simulink model "KalmanFIlter"  (R2022b)
settings: Solver=VariableStepAuto  StartTime=0.0  StopTime=timetorevolve  RelTol=1e-3
model workspace (MAT data in the model file):
  Ts_Camera = 0.1
values from neighbouring files (symbols this model uses):
  ConstantO = 2*pi/(timetorevolve)    (= 0.00118999721727)    [SystemVariables.m]
  Ts_System = 1/system_Frequency    (= 0.1)    [SystemVariables.m]
libraries: robotcorelib x3, simulink x1
settings Model: Creator=Xamza  LastModifiedBy=Xamza

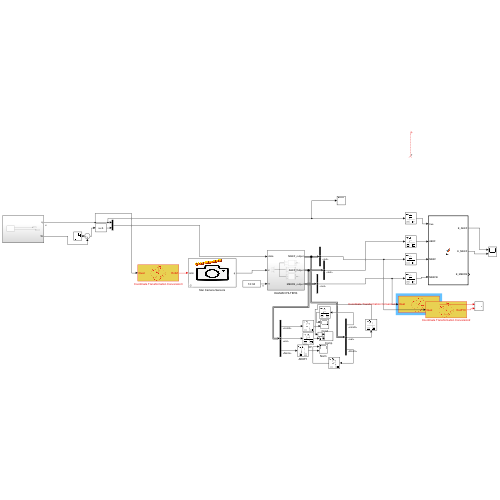
[thumbnail: Simulink's stored preview of the top-level diagram]
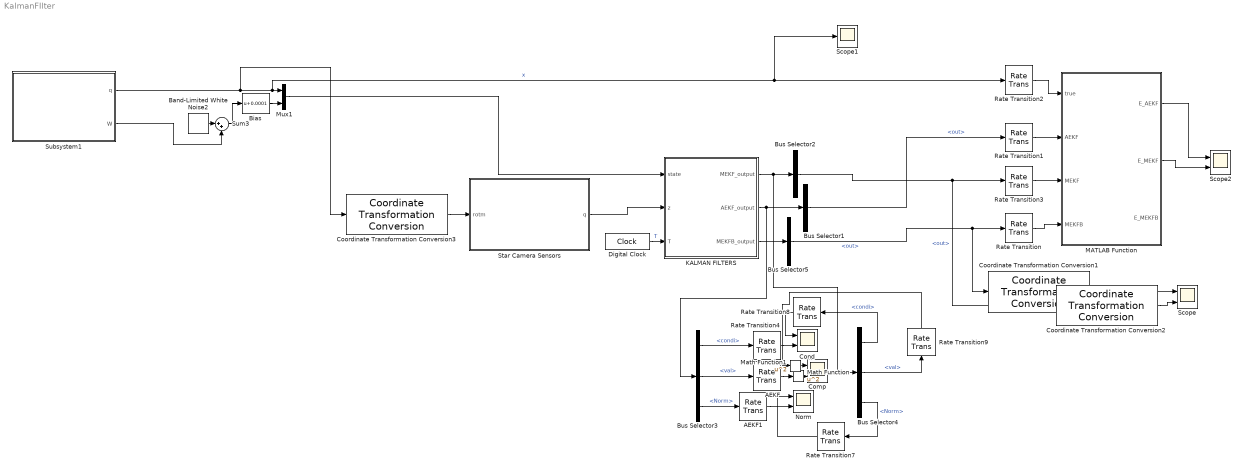
== system KalmanFIlter ==
  AEKF : RateTransition  Integrity=off  OutPortSampleTime=ComTs
  AEKF1 : RateTransition  Integrity=off  OutPortSampleTime=ComTs
  Band-Limited White Noise2 : simulink/Sources/Band-Limited White Noise  Cov=[0.00001]  Ts=Ts_System  seed=[23341]
  Bias : Bias  Bias=0.0001  SaturateOnIntegerOverflow=off
  Bus Selector1 : BusSelector  OutputSignals=out
  Bus Selector2 : BusSelector  OutputSignals=out
  Bus Selector3 : BusSelector  OutputSignals=condi,val,Norm
  Bus Selector4 : BusSelector  OutputSignals=condi,val,Norm
  Bus Selector5 : BusSelector  OutputSignals=out
  Comp : Scope  NumInputPorts=2
  Cond : Scope  NumInputPorts=2
  Coordinate Transformation Conversion1 : robotcorelib/Coordinate Transformation Conversion  InputRepresentation=Quaternion  InputEulerSequence=ZYX  ShowTrVecInputPort=on  OutputRepresentation=Euler Angles  OutputEulerSequence=ZYX  ShowTrVecOutputPort=on  SimulateUsing=Interpreted execution
  Coordinate Transformation Conversion2 : robotcorelib/Coordinate Transformation Conversion  InputRepresentation=Quaternion  InputEulerSequence=ZYX  ShowTrVecInputPort=on  OutputRepresentation=Euler Angles  OutputEulerSequence=ZYX  ShowTrVecOutputPort=on  SimulateUsing=Interpreted execution
  Coordinate Transformation Conversion3 : robotcorelib/Coordinate Transformation Conversion  InputRepresentation=Quaternion  InputEulerSequence=ZYX  ShowTrVecInputPort=on  OutputRepresentation=Rotation Matrix  OutputEulerSequence=ZYX  ShowTrVecOutputPort=on  SimulateUsing=Interpreted execution
  Digital Clock : DigitalClock  SampleTime=Ts_System
  KALMAN FILTERS : Subsystem
  MATLAB Function : MATLAB Function  TreatAsAtomicUnit=on
  Math Function : Math  Operator=square
  Math Function1 : Math  Operator=square
  Mux1 : Mux  Inputs=2
  Norm : Scope  NumInputPorts=2
  Rate Transition{,1..4,7..9} (8 alike) : RateTransition  Integrity=off  OutPortSampleTime=ComTs
  Scope : Scope  NumInputPorts=2
  Scope1 : Scope
  Scope2 : Scope  NumInputPorts=2
  Star Camera Sensors : Subsystem  mask{StarOne=on, StarTwo=on, StarThree=on, StarFour=on, StarFive=on, StarSix=on}
      mask prompts: StarOne "Star Camera One"; StarTwo "Star Camera Two"; StarThree "Star Camera Three"; StarFour "Star Camera Four"; StarFive "Star Camera Five"; StarSix "Star Camera Six"
      mask DialogControl DescGroupVar Prompt: Star Camera Settings
      mask DialogControl ParameterGroupVar Prompt: Available Star Cameras
      mask Display: image('$imagefile'); % Use "Edit Image" on toolstrip to change.
  Subsystem1 : Subsystem
  Sum3 : Sum  Inputs=|++
  wires:
  Coordinate Transformation Conversion3/1 -> Star Camera Sensors/1(rotm)
  Star Camera Sensors/1(q) -> KALMAN FILTERS/2(z)
  ? -> ?  "T"
  Sum3/1 -> Bias/1
  Subsystem1/1(q) -> Scope1/1, Rate Transition2/1, Mux1/1, Coordinate Transformation Conversion3/1  "x"
  Subsystem1/2(W) -> Sum3/2
  Band-Limited White Noise2/1 -> Sum3/1
  MATLAB Function/1(E_AEKF) -> Scope2/1
  MATLAB Function/2(E_MEKF) -> Scope2/2
  Rate Transition/1 -> MATLAB Function/4(MEKFB)
  Rate Transition1/1 -> MATLAB Function/2(AEKF)
  Rate Transition2/1 -> MATLAB Function/1(true)
  Mux1/1 -> KALMAN FILTERS/1(state)
  Digital Clock/1 -> KALMAN FILTERS/3(T)  "T"
  KALMAN FILTERS/2(AEKF_output) -> Bus Selector3/1, Bus Selector1/1
  KALMAN FILTERS/3(MEKFB_output) -> Bus Selector5/1
  Bus Selector3/1 -> Rate Transition4/1  "<condi>"
  Bus Selector3/3 -> AEKF1/1  "<Norm>"
  Bus Selector3/2 -> AEKF/1  "<val>"
  KALMAN FILTERS/1(MEKF_output) -> Bus Selector2/1, Bus Selector4/1
  Bus Selector4/1 -> Rate Transition8/1  "<condi>"
  Bus Selector4/2 -> Rate Transition9/1  "<val>"
  Bus Selector4/3 -> Rate Transition7/1  "<Norm>"
  Bias/1 -> Mux1/2
  Bus Selector5/1 -> Rate Transition/1, Coordinate Transformation Conversion1/1  "<out>"
  Rate Transition3/1 -> MATLAB Function/3(MEKF)
  Bus Selector1/1 -> Rate Transition1/1  "<out>"
  Bus Selector2/1 -> Rate Transition3/1, Coordinate Transformation Conversion2/1  "<out>"
  Rate Transition4/1 -> Cond/2
  AEKF1/1 -> Norm/2
  Rate Transition7/1 -> Norm/1
  Rate Transition8/1 -> Cond/1
  Rate Transition9/1 -> Math Function1/1
  AEKF/1 -> Math Function/1
  Math Function/1 -> Comp/2
  Math Function1/1 -> Comp/1
  Coordinate Transformation Conversion1/1 -> Scope/1
  Coordinate Transformation Conversion2/1 -> Scope/2

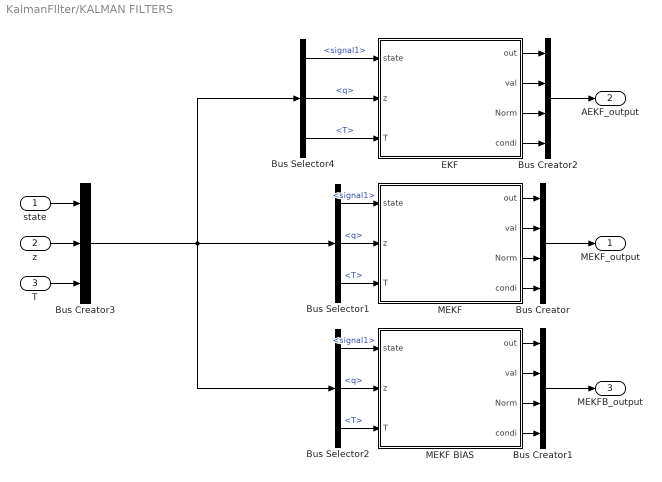
== system KalmanFIlter/KALMAN FILTERS ==
  state : Inport
  z : Inport  Port=2
  T : Inport  Port=3
  Bus Creator : BusCreator  Inputs=4
  Bus Creator1 : BusCreator  Inputs=4
  Bus Creator2 : BusCreator  Inputs=4
  Bus Creator3 : BusCreator  Inputs=3
  Bus Selector1 : BusSelector  OutputSignals=signal1,q,T
  Bus Selector2 : BusSelector  OutputSignals=signal1,q,T
  Bus Selector4 : BusSelector  OutputSignals=signal1,q,T
  EKF : MATLAB Function  TreatAsAtomicUnit=on
  MEKF : MATLAB Function  TreatAsAtomicUnit=on
  MEKF BIAS : MATLAB Function  TreatAsAtomicUnit=on
  MEKF_output : Outport
  AEKF_output : Outport  Port=2
  MEKFB_output : Outport  Port=3
  wires:
  Bus Creator2/1 -> AEKF_output/1
  MEKF/1(out) -> Bus Creator/1
  MEKF/2(val) -> Bus Creator/2
  MEKF/3(Norm) -> Bus Creator/3
  MEKF/4(condi) -> Bus Creator/4
  Bus Creator/1 -> MEKF_output/1
  MEKF BIAS/1(out) -> Bus Creator1/1
  MEKF BIAS/2(val) -> Bus Creator1/2
  MEKF BIAS/3(Norm) -> Bus Creator1/3
  MEKF BIAS/4(condi) -> Bus Creator1/4
  Bus Creator1/1 -> MEKFB_output/1
  EKF/1(out) -> Bus Creator2/1
  EKF/2(val) -> Bus Creator2/2
  EKF/3(Norm) -> Bus Creator2/3
  EKF/4(condi) -> Bus Creator2/4
  state/1 -> Bus Creator3/1
  z/1 -> Bus Creator3/2
  T/1 -> Bus Creator3/3
  Bus Creator3/1 -> Bus Selector4/1, Bus Selector2/1, Bus Selector1/1
  Bus Selector4/1 -> EKF/1(state)  "<signal1>"
  Bus Selector4/2 -> EKF/2(z)  "<q>"
  Bus Selector4/3 -> EKF/3(T)  "<T>"
  Bus Selector1/3 -> MEKF/3(T)  "<T>"
  Bus Selector2/2 -> MEKF BIAS/2(z)  "<q>"
  Bus Selector2/1 -> MEKF BIAS/1(state)  "<signal1>"
  Bus Selector2/3 -> MEKF BIAS/3(T)  "<T>"
  Bus Selector1/1 -> MEKF/1(state)  "<signal1>"
  Bus Selector1/2 -> MEKF/2(z)  "<q>"

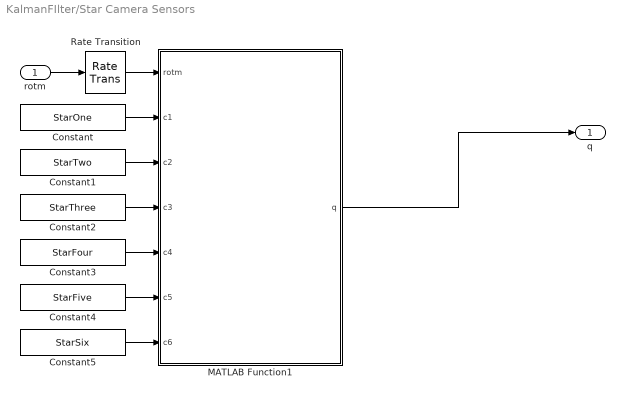
== system KalmanFIlter/Star Camera Sensors ==
  rotm : Inport
  Constant : Constant  Value=StarOne
  Constant1 : Constant  Value=StarTwo
  Constant2 : Constant  Value=StarThree
  Constant3 : Constant  Value=StarFour
  Constant4 : Constant  Value=StarFive
  Constant5 : Constant  Value=StarSix
  MATLAB Function1 : MATLAB Function  TreatAsAtomicUnit=on
  Rate Transition : RateTransition  Integrity=off  OutPortSampleTime=Ts_Camera
  q : Outport
  wires:
  MATLAB Function1/1(q) -> q/1
  rotm/1 -> Rate Transition/1
  Constant1/1 -> MATLAB Function1/3(c2)
  Constant/1 -> MATLAB Function1/2(c1)
  Constant5/1 -> MATLAB Function1/7(c6)
  Constant4/1 -> MATLAB Function1/6(c5)
  Constant3/1 -> MATLAB Function1/5(c4)
  Constant2/1 -> MATLAB Function1/4(c3)
  Rate Transition/1 -> MATLAB Function1/1(rotm)

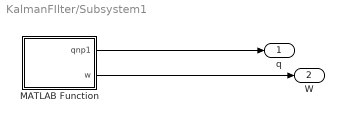
== system KalmanFIlter/Subsystem1 ==
  MATLAB Function : MATLAB Function  TreatAsAtomicUnit=on
  q : Outport
  W : Outport  Port=2
  wires:
  MATLAB Function/2(w) -> W/1
  MATLAB Function/1(qnp1) -> q/1

== matlab function KalmanFIlter/Star Camera Sensors/MATLAB Function1 ==
  data: rotm input; q output; c1 input; c2 input; c3 input; c4 input; c5 input; c6 input
function q  = fcn(rotm,c1,c2,c3,c4,c5,c6)
pose=rotm2eul(rotm);
persistent Cam1 Cam2 Cam3 Cam4 Cam5 Cam6
for i=1
if isempty(Cam1)
stars=100;
Star_Base=zeros(3,stars);
for i=1:stars
    v=[rand*randi([-5 5],1);rand*randi([-5 5],1);rand*randi([-5 5],1)];
Star_Base(:,i)=v/norm(v);
end 

map=Star_Base;

C1_R=eul2rotm([0,0,0]);
C2_R=eul2rotm([0,0,pi/2],'XYZ');
C3_R=eul2rotm([0,0,-pi],'XYZ');
C4_R=eul2rotm([0,0,-pi/2],'XYZ');
C5_R=eul2rotm([0,-pi/2,0],'XYZ');
C6_R=eul2rotm([0,pi/2,0],'XYZ');    
Cam1=StarCamera(C1_R,70,map);
Cam2=StarCamera(C2_R,70,map);
Cam3=StarCamera(C3_R,70,map);
Cam4=StarCamera(C4_R,70,map);
Cam5=StarCamera(C5_R,70,map);
Cam6=StarCamera(C6_R,70,map);
q=[1;0;0;0;];

end


end

Cam1.IsTurnedOn=c1;
Cam2.IsTurnedOn=c2;
Cam3.IsTurnedOn=c3;
Cam4.IsTurnedOn=c4;
Cam5.IsTurnedOn=c5;
Cam6.IsTurnedOn=c6;


sensorState=[Cam1.IsTurnedOn;Cam2.IsTurnedOn;Cam3.IsTurnedOn;Cam4.IsTurnedOn;Cam5.IsTurnedOn;Cam6.IsTurnedOn];
idx=find(sensorState>0);    

q1=(Cam1.DevanportQ(pose)')';
q2=(Cam2.DevanportQ(pose)')';
q3=(Cam3.DevanportQ(pose)')';
q4=(Cam4.DevanportQ(pose)')';
q5=(Cam5.DevanportQ(pose)')';
q6=(Cam6.DevanportQ(pose)')';


qs=[q1,q2,q3,q4,q5,q6];
q=real(AverageQuaternion(real(qs(:,idx))));
if isempty(idx)
    q=[999*i;0;0;0];
end

== matlab function KalmanFIlter/KALMAN FILTERS/EKF ==
  settings: updateMethod=DISCRETE  sampleTime=Ts_System
  data: state input; z input; Ts_System parameter; out output; Ts_Camera parameter; T input; val output; Norm output; condi output
function [out,val,Norm,condi]= fcn(state,z, Ts_System, Ts_Camera,T)
persistent  P Q Rn x
tic
if isempty(Q)
    P = 0.1*eye(4);
    Q = 10*eye(4);
    Rn = 0.1*eye(4);
    x=state(1:4);
end


w=state(5:end);
A=Amatrix(w(1),w(2),w(3),Ts_System);
%C=Cmatrix2(z(1),z(2),z(3),z(4));
C=eye(4);
% EKF
%%Prediction
x_hat = A*x;
x_hat=x_hat/norm(x_hat);
p_hat = A*P*A' + Q;
if z(1)<999 & mod(T,Ts_Camera)==0 
%%update
y = C*abs(z)-C*abs(x_hat);

S = C*P*C'+Rn;
K = P*C'*inv(S);
x = x_hat + K*y;
x = x/norm(x);
out=x;
P = (eye(4) - (K*C))*p_hat;
else
x=x_hat/norm(x_hat);
out=x;
P=p_hat;
end
val=toc;
disp("AEKF")
Norm=norm(P)
disp("AEKF")
condi=cond(P);

end

== matlab function KalmanFIlter/KALMAN FILTERS/MEKF ==
  settings: updateMethod=DISCRETE  sampleTime=Ts_System
  data: state input; z input; Ts_System parameter; out output; val output; Ts_Camera parameter; T input; Norm output; condi output
function [out,val,Norm,condi] = fcn(state,z, Ts_System, Ts_Camera,T)
persistent  P Rn x A q_ref
   
if isempty(P)
    P = 0.0001*eye(3);
    Rn = 0.01*eye(3);
    x=[0,0,0]';
    q_ref=state(1:4);


end
tic
Q=Qmatrix(Ts_System);
Q=Q(1:3,1:3);
G=[-eye(3)];
H=[eye(3)];

%%Prediction

w=state(5:end);
q_pred=Amatrix(w(1),w(2),w(3),Ts_System)*q_ref;
wx=[0 -w(3) w(2);
    w(3) 0 -w(1);
   -w(2) w(1) 0];
F=[-wx];
F = (eye(3)+F*Ts_System);
F=Fmatrix(Ts_System,w);
F=F(1:3,1:3);
p_hat=F*P*F'+G*Q*G';
if z(1)<999 & mod(T,Ts_Camera)==0 
%%update
S = H*p_hat*H'+Rn;
K = p_hat*H'*inv(S);

qe = flip(quadprod((z),quatinverse(q_pred)));
am=(qe(1:3)/qe(4));
%am=qe(1:3)/(1+qe(4));
x=K*am;

P = (eye(3) - (K*H))*p_hat;

else
x(1:3)=zeros(3,1);
P=p_hat;
end
w=w;
dq=flip([x(1:3);2]/norm([x(1:3);2]));
q_pred=q_pred+Amatrix(w(1),w(2),w(3),Ts_System)*quadprod(dq,q_ref);
q_pred=(q_pred/norm(q_pred));
out=q_pred;
x=zeros(3,1);
q_ref=q_pred;
val=toc;
disp("MEKF")
Norm=norm(P)
disp("MEKF")
condi=cond(P);

== matlab function KalmanFIlter/MATLAB Function ==
  data: true input; AEKF input; MEKF input; E_AEKF output; MEKFB input; E_MEKF output; E_MEKFB output
function [E_AEKF,E_MEKF,E_MEKFB] = fcn(true,AEKF,MEKF,MEKFB)

true=abs(true);
AEKF=abs(AEKF);
MEKF=(abs(MEKF));
E_MEKF=sqrt(norm(true-MEKF));
E_MEKFB=(norm(true-MEKFB));
E_AEKF=sqrt(norm(true-AEKF));

== matlab function KalmanFIlter/Subsystem1/MATLAB Function ==
  data: qnp1 output; w output; Ts_System parameter; ConstantO parameter
function [qnp1,w]= fcn(Ts_System, ConstantO)
persistent q  

if isempty(q)
v=[1,1,1,1];
q=(v/norm(v))';
end



c=ConstantO;
w=[0,1,0]'*c;
qnp1=Amatrix(w(1),w(2),w(3),Ts_System)*q;
qnp1=qnp1/norm(qnp1);
q=qnp1;

== matlab function KalmanFIlter/KALMAN FILTERS/MEKF BIAS ==
  settings: updateMethod=DISCRETE  sampleTime=Ts_System
  data: state input; z input; Ts_System parameter; out output; val output; Ts_Camera parameter; T input; Norm output; condi output
function [out,val,Norm,condi] = fcn(state,z, Ts_System, Ts_Camera,T)
persistent  P Rn x A q_ref B
   
if isempty(P)
    P = 0.1*eye(6);
    B=zeros(3,1)*0.1;
    Rn = 0.01*eye(3);
    x=[0,0,0,0,0,0]';
    q_ref=state(1:4);


end
tic
Q=Qmatrix(Ts_System);
G=[-eye(3) zeros(3);zeros(3) eye(3)];
H=[eye(3),zeros(3,3)];

%%Prediction

w=state(5:end)-B;
q_pred=Amatrix(w(1),w(2),w(3),Ts_System)*q_ref;
wx=[0 -w(3) w(2);
    w(3) 0 -w(1);
   -w(2) w(1) 0];

F=Fmatrix(Ts_System,w);
F=[wx -eye(3);zeros(3,3),zeros(3,3)];
F = (eye(6)+F*Ts_System);
p_hat=F*P*F'+G*Q*G';
if z(1)<999 & mod(T,Ts_Camera)==0 
%%update
S = H*p_hat*H'+Rn;
K = p_hat*H'*inv(S);

qe = flip(quadprod((z),quatinverse(q_pred)));
am=(qe(1:3)/qe(4));
%am=qe(1:3)/(1+qe(4));
x=K*am;
P = (eye(6) - (K*H))*p_hat;
B=B+x(4:6);
else
x(1:3)=zeros(3,1);
P=p_hat;
end
w=w-x(4:6);

dq=flip([x(1:3);2]/norm([x(1:3);2]));
q_pred=q_pred+Amatrix(w(1),w(2),w(3),Ts_System)*quadprod(dq,q_ref);
q_pred=(q_pred/norm(q_pred));
out=q_pred;
x=zeros(6,1);
q_ref=q_pred;
val=1/toc;
Norm=norm(P);
condi=cond(P);
